simulink model "simplified_sim_for_linearize"  (R2024b)
settings: Solver=VariableStepAuto  StartTime=0.0  StopTime=15  FixedStep=0.05  MaxStep=0.2  RelTol=1e-3
values from neighbouring files (symbols this model uses):
  AfoilA = 0.046    [model_parameters.m]
  AfoilFP = 0.048    [model_parameters.m]
  AfoilFS = 0.048    [model_parameters.m]
  alpha0012 = data0012(:,1)    [model_parameters.m]
  alpha63412wing = data63412wing(:,1)    [model_parameters.m]
  cd0012 = data0012(:,3)    [model_parameters.m]
  cdi63412wing = data63412wing(:,4)    [model_parameters.m]
  cdv63412wing = data63412wing(:,5)    [model_parameters.m]
  cl63412wing = data63412wing(:,3)    [model_parameters.m]
  cm63412wing = data63412wing(:,9)    [model_parameters.m]
  csA = 0.1    [model_parameters.m]
  csF = 0.08    [model_parameters.m]
  foilA_ARM = [-dxa, dya, dza]    [model_parameters.m]
  foilFP_ARM = [dxf, -dyf, dzf]    [model_parameters.m]
  foilFS_ARM = [dxf, dyf, dzf]    [model_parameters.m]
  g = 9.81    [model_parameters.m]
  LAd = 0.08*pi*(0.8)^3/64    (= 0.0020106192983)    [model_parameters.m]
  LFPd = integral(fpint, foilFP_ARM(2)-0.4, foilFP_ARM(2)+0.4)    [model_parameters.m]
  LFSd = integral(fsint, foilFS_ARM(2)-0.4, foilFS_ARM(2)+0.4)    [model_parameters.m]
  M_RB_1 = inv(M_RB)    [dimensionalize_model.m]    (also in model_parameters.m = M_RB^(-1))
  MAC_A = 0.08    [model_parameters.m]
  MAC_FP = 0.08    [model_parameters.m]
  MAC_FS = 0.08    [model_parameters.m]
  mass = 215    [dimensionalize_model.m]    (also in model_parameters.m)
  propwake = 0.05    [model_parameters.m]
  r_g = [0; 0; 0]    [dimensionalize_model.m]    (also in model_parameters.m = [xg, yg, zg])
  rho = 1024.8    [model_parameters.m]
  spanA = 0.76    [model_parameters.m]
  spanFP = 0.76    [model_parameters.m]
  spanFS = 0.76    [model_parameters.m]
  tA = 0.12*0.08    (= 0.0096)    [model_parameters.m]
  tFP = 0.12*0.08    (= 0.0096)    [model_parameters.m]
  tFS = 0.12*0.08    (= 0.0096)    [model_parameters.m]
  usted = 7    [model_parameters.m]
  wagC1 = 0.165    [model_parameters.m]
  wagC2 = 0.335    [model_parameters.m]
  wage1 = 0.0455*(usted/(MAC_FP/2))    (= 7.9625)    [model_parameters.m]
  wage2 = 0.3*(usted/(MAC_FP/2))    (= 52.5)    [model_parameters.m]
  zpr = dza    (= 0.96)    [model_parameters.m]
undefined symbols (not defined in the file or in its folder): magnitude
libraries: mssSimulink x11, matrix_library x3, simulink_extras x3
(part 2 of 2)

== matlab function simplified_sim_for_linearize/Hydrofoil Craft/Hydrofoil Forces/Hydrofoil [A]/CP ==
  data: lx output; ly output; ac input; lz output; foil_arm input
function [lx,ly,lz] = CP_HSF(ac, foil_arm)
% This function will calculate the moment arm for the center of 
% pressure of a hydrofoil based on control deflection. 
% Used when the pivot point is different from the center of pressure, and
% set to the original foil CP defined in the params otherwise.



lx = foil_arm(1);
ly = foil_arm(2);
lz = foil_arm(3);

== matlab function simplified_sim_for_linearize/Hydrofoil Craft/Hydrofoil Forces/Hydrofoil [FS]/STRUT FP/lateralDamp ==
  data: h_sub input; strutK output; zs input; V input; p input; cs input; rho parameter
function strutK = strutrolldamp(h_sub, zs, V, p, cs, rho)

strutK = -0.5*rho*V*2*pi*p*cs*(zs.^3-(zs+0.1-h_sub).^3)*(1/3);

== matlab function simplified_sim_for_linearize/Hydrofoil Craft/Hydrofoil Forces/Hydrofoil [A]/Foil Theory/AdditionalDrag/Additional Drag ==
  data: cdind input; dinc output; span input; hsub input; t input; c input; cdw output; cdint output; usted parameter
function [dinc, cdw, cdint]   = addedDrag(cdind, span, hsub, t, c, usted)

%V = 7m/s not very correct in general 
hsub = abs(hsub);
dinc = (2-(33*(hsub/span)^(3/2))/(33*(hsub/span)^(3/2)+1))*cdind;
frh = usted/sqrt(9.81*hsub);
cdw = 1/(2*frh^2)*(c/hsub)*exp(-2/frh^2);
cdint = 0.75*(t/c)-0.0003*(t/c)^(-2);

== matlab function simplified_sim_for_linearize/Hydrofoil Craft/Gravitational Forces ==
  data: euler_angles input; g_tau output; mass parameter; g parameter; r_g parameter
function g_tau = Gravity(euler_angles, mass, g, r_g)


phi = euler_angles(1);
theta = euler_angles(2);
psy = euler_angles(3);

% m*g * z[NED] expressed in BF through DCM [BF]C[NED]

Xg = -mass*g*sin(theta);
Yg = mass*g*cos(theta)*sin(phi);
Zg = mass*g*cos(theta)*cos(phi);

Kg = r_g(2)*mass*g*cos(theta)*cos(phi) - r_g(3)*mass*g*cos(theta)*sin(phi);
Mg = -r_g(3)*mass*g*sin(theta)-r_g(1)*mass*g*cos(theta)*cos(phi);
Ng = r_g(1)*mass*g*cos(theta)*sin(phi) + r_g(2)*mass*g*sin(theta);

g_tau = [Xg; Yg; Zg; Kg; Mg; Ng];

== matlab function simplified_sim_for_linearize/Hydrofoil Craft/Hydrofoil Forces/Hydrofoil [FP]/CP ==
  data: lx output; ly output; ac input; lz output; foil_arm input
function [lx,ly,lz] = CP_HSF(ac, foil_arm)
% This function will calculate the moment arm for the center of 
% pressure of a hydrofoil based on control deflection. 
% Used when the pivot point is different from the center of pressure, and
% set to the original foil CP defined in the params otherwise.



lx = foil_arm(1);
ly = foil_arm(2);
lz = foil_arm(3);

== matlab function simplified_sim_for_linearize/Hydrofoil Craft/Hydrofoil Forces/Hydrofoil [FP]/Foil Theory/AdditionalDrag/Additional Drag ==
  data: cdind input; dinc output; span input; hsub input; t input; c input; cdw output; cdint output; usted parameter
function [dinc, cdw, cdint]   = addedDrag(cdind, span, hsub, t, c, usted)

%V = 7m/s not very correct in general 
hsub = abs(hsub);
dinc = (2-(33*(hsub/span)^(3/2))/(33*(hsub/span)^(3/2)+1))*cdind;
frh = usted/sqrt(9.81*hsub);
cdw = 1/(2*frh^2)*(c/hsub)*exp(-2/frh^2);
cdint = 0.75*(t/c)-0.0003*(t/c)^(-2);

== matlab function simplified_sim_for_linearize/Hydrofoil Craft/Hydrofoil Forces/Hydrofoil [FP]/Force and Moment Calculation ==
  data: L input; D input; FX output; ainf input; FY output; FZ output; Marm input; MX output; MY output; MZ output
function [FX, FY, FZ, MX, MY, MZ] = HydrodynamicForces(L, D, ainf, Marm)


%%%%%%%%% ----------------- %%%%%%%%

% Vrel is :
% u+qz-ry  
% v+rx-pz
% w+py-qx

%Inflow velocity is this vector's magnitude, however, in 2D analysis,
%considering the y direction velocity will lead to issues. Change this if
%needed for lateral dynamics!

%Vinf_s is squared already
Rbh = [cos(ainf) 0 -sin(ainf);0 1 0;sin(ainf) 0 cos(ainf)];

forces = Rbh*[-D; 0; -L]; %Only Longitudinal Dynamics
[FX, FY, FZ] = deal(forces(1), forces(2), forces(3));
moments = cross(Marm,[FX, FY, FZ]);
[MX, MY, MZ] = deal(moments(1), moments(2), moments(3));

== matlab function simplified_sim_for_linearize/Hydrofoil Craft/Hydrofoil Forces/Hydrofoil [FP]/STRUT FP/lateralDamp ==
  data: h_sub input; strutK output; zs input; V input; p input; cs input; rho parameter
function strutK = strutrolldamp(h_sub, zs, V, p, cs, rho)

strutK = -0.5*rho*V*2*pi*p*cs*(zs.^3-(zs+0.1-h_sub).^3)*(1/3);
